simulink model "pruebas_Frec_Imax"  (R2023b)
settings: Solver=VariableStepAuto  StartTime=0.0  StopTime=10.0  MaxStep=0.001  RelTol=1e-3
libraries: simulink x2
settings Model: Creator=USUARIO  LastModifiedBy=USUARIO

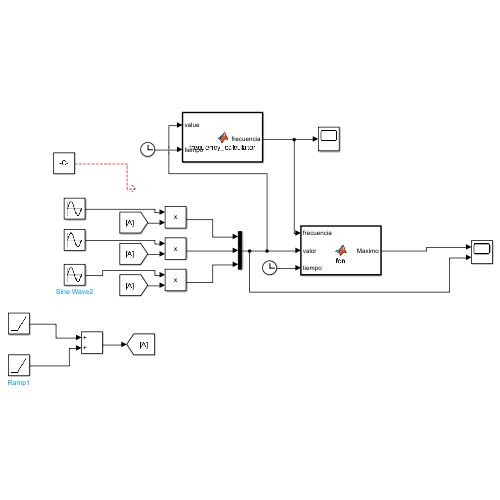
[thumbnail: Simulink's stored preview of the top-level diagram]
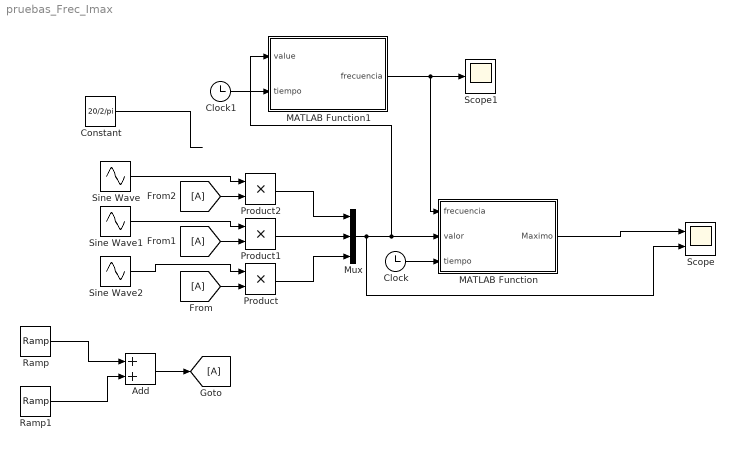
== system pruebas_Frec_Imax ==
  Add : Sum
  Clock : Clock
  Clock1 : Clock
  Constant : Constant  Value=20/2/pi
  From : From
  From1 : From
  From2 : From
  Goto : Goto
  MATLAB Function : MATLAB Function  TreatAsAtomicUnit=on
  MATLAB Function1 : MATLAB Function  TreatAsAtomicUnit=on
  Mux : Mux  Inputs=3
  Product : Product
  Product1 : Product
  Product2 : Product
  Ramp : simulink/Sources/Ramp  slope=1  start=1  InitialOutput=0
  Ramp1 : simulink/Sources/Ramp  slope=-3  start=5  InitialOutput=0
  Scope : Scope  NumInputPorts=2
  Scope1 : Scope
  Sine Wave : Sin  Frequency=20  SampleTime=0
  Sine Wave1 : Sin  Frequency=20  Phase=+2/3*pi  SampleTime=0
  Sine Wave2 : Sin  Frequency=20  Phase=-2/3*pi  SampleTime=0
  wires:
  Ramp/1 -> Add/1
  Ramp1/1 -> Add/2
  Add/1 -> Goto/1
  Sine Wave1/1 -> Product1/1
  Sine Wave/1 -> Product2/1
  Sine Wave2/1 -> Product/1
  Mux/1 -> Scope/2, MATLAB Function1/1(value), MATLAB Function/2(valor)
  From/1 -> Product/2
  From1/1 -> Product1/2
  From2/1 -> Product2/2
  Product1/1 -> Mux/2
  Product/1 -> Mux/3
  Product2/1 -> Mux/1
  Constant/1 -> ?
  Clock/1 -> MATLAB Function/3(tiempo)
  MATLAB Function/1(Maximo) -> Scope/1
  Clock1/1 -> MATLAB Function1/2(tiempo)
  MATLAB Function1/1(frecuencia) -> MATLAB Function/1(frecuencia), Scope1/1

== matlab function pruebas_Frec_Imax/MATLAB Function1 ==
  settings: updateMethod=DISCRETE
  data: frecuencia output; value input; tiempo input
function frecuencia = frecuency_calculator(value,tiempo)

   persistent signo
    if isempty(signo)
       signo=[0 0 0]; % 1 positive, 2 negative
    end
    persistent t_inicio
    if isempty(t_inicio)
       t_inicio=[0 0 0];
    end

    persistent frecuencia_acc
    if isempty(frecuencia_acc)
       frecuencia_acc=1;
    end

    frecuencia=frecuencia_acc;

    for i=1:3
    
        if signo(i) == 0
            if value(i) >= 0 
                signo(i) = 1;
            else
                signo(i) = 2;
            end
            t_inicio(i)=tiempo;
        end
        
        if signo(i)==1
            if value(i) <= 0
                frecuencia = 1/(2*(tiempo-t_inicio(i)));
                frecuencia_acc=frecuencia;
                signo(i) = 0;
            end
        end
        
        if signo(i)==2
            if value(i) >= 0
                frecuencia = 1/(2*(tiempo-t_inicio(i)));
                frecuencia_acc=frecuencia;
                signo(i) = 0;
            end
        end

    end

== matlab function pruebas_Frec_Imax/MATLAB Function ==
  settings: updateMethod=DISCRETE
  data: frecuencia input; Maximo output; valor input; tiempo input
function Maximo = fcn(frecuencia,valor,tiempo)

   persistent antiguo_maximo
    if isempty(antiguo_maximo)
       antiguo_maximo=0;
    end
    persistent t_maximo
    if isempty(t_maximo)
       t_maximo=0;
    end

maximo = [0 0 0];

periodo=1/abs(frecuencia)/3;

for i=1:3
    if abs(valor(i))>=antiguo_maximo
        maximo(i)=abs(valor(i));
        antiguo_maximo=abs(valor(i));
        t_maximo=tiempo;
    else
        maximo(i)=antiguo_maximo;
        if tiempo>t_maximo+periodo
            maximo(i)=abs(valor(i));
            antiguo_maximo=abs(valor(i));
            t_maximo=tiempo;
        end
    end
end

Maximo = max(maximo);
